simulink model "center_tapped_RL_high"  (R2022b)
settings: Solver=VariableStepAuto  StartTime=0.0  StopTime=00.1  RelTol=1e-3
libraries: spsCurrentMeasurementLib x3, spsVoltageMeasurementLib x3, spsDiodeLib x2, spsACVoltageSourceLib x1, spsLinearTransformerLib x1, spsSeriesRLCBranchLib x1, sps_lib x1
settings Model: Creator=mroun  LastModifiedBy=mroun

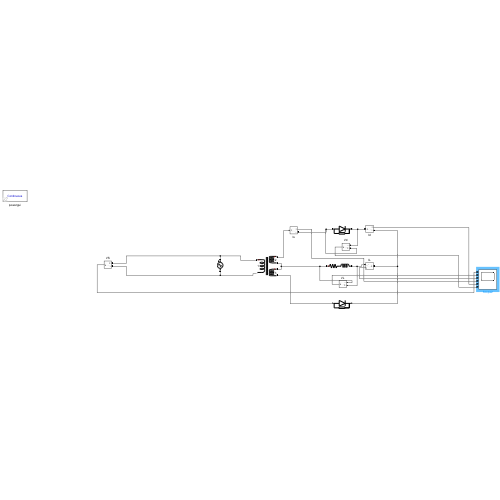
[thumbnail: Simulink's stored preview of the top-level diagram]
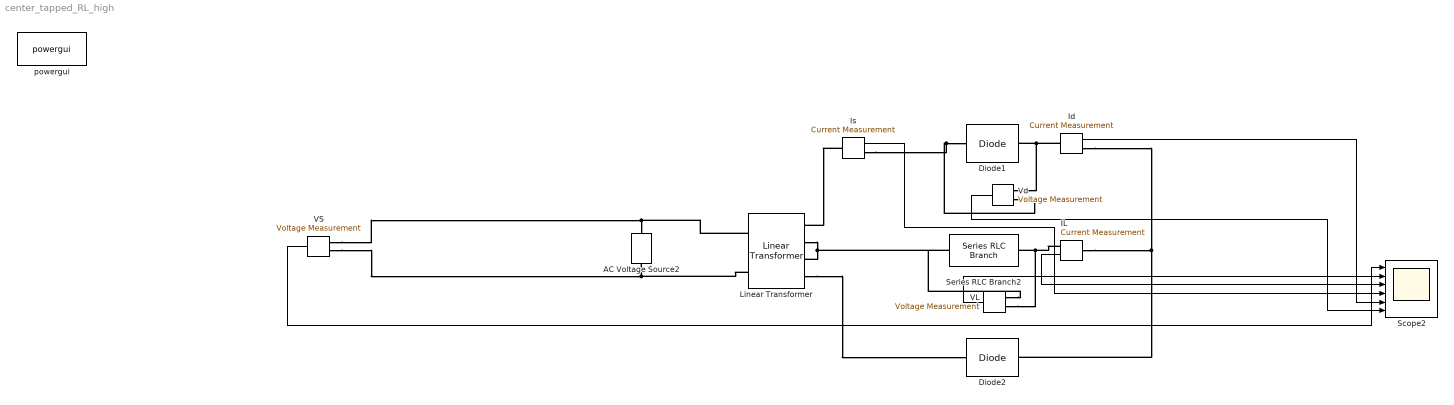
== system center_tapped_RL_high ==
  AC Voltage Source2 : spsACVoltageSourceLib/AC Voltage Source  Amplitude=200  Phase=0  Frequency=50  SampleTime=0  Measurements=None  BusType=swing  Pref=10e3  Qref=0  Qmin=-inf  Qmax=+inf
  Diode1 : spsDiodeLib/Diode  Ron=0.001  Lon=0  Vf=0.8  IC=0  UseSnubber=0  Rs=500  Cs=250e-9  Measurements=off
  Diode2 : spsDiodeLib/Diode  Ron=0.001  Lon=0  Vf=0.8  IC=0  UseSnubber=0  Rs=500  Cs=250e-9  Measurements=off
  IL : spsCurrentMeasurementLib/Current Measurement  PhasorSimulation=off  OutputType=Complex  PSBequivalent=0
  Id : spsCurrentMeasurementLib/Current Measurement  PhasorSimulation=off  OutputType=Complex  PSBequivalent=0
  Is : spsCurrentMeasurementLib/Current Measurement  PhasorSimulation=off  OutputType=Complex  PSBequivalent=0
  Linear Transformer : spsLinearTransformerLib/Linear Transformer  UNITS=pu  NominalPower=[ 1e3 50 ]  winding1="[ 200  0.002  0.08 ]"  winding2="[ 100  0.002  0.08 ]"  ThreeWindings=on  winding3=[ 100 0.002 0.08 ]  RmLm=[ 2 1 ]  Measurements=None  DataType=off
  Scope2 : Scope  NumInputPorts=6
  Series RLC Branch2 : spsSeriesRLCBranchLib/Series RLC Branch  LConnTagsString=__new0  RConnTagsString=__new0  BranchType=RL  Resistance=10  Inductance=1  SetiL0=off  InitialCurrent=2  Capacitance=1e-6  Setx0=off  InitialVoltage=0  Measurements=None
  VL : spsVoltageMeasurementLib/Voltage Measurement  PhasorSimulation=off  OutputType=Complex  PSBequivalent=0
  VS : spsVoltageMeasurementLib/Voltage Measurement  PhasorSimulation=off  OutputType=Complex  PSBequivalent=0
  Vd : spsVoltageMeasurementLib/Voltage Measurement  PhasorSimulation=off  OutputType=Complex  PSBequivalent=0
  powergui : sps_lib/powergui  Priority=1  SimulationMode=Continuous  SampleTime=50e-6  frequency=60  Iterations=50  frequencyindice=50  Pbase=100e6  ErrMax=1e-4  UnitsV=kV  UnitsW=MW  buscounter=0  FunctionMessages=off  echomessages=off  EnableUseOfTLC=off  CurrentSourceSwitches=off  DisableSnubberDevices=off  DisableRonSwitches=off  DisableVfSwitches=off  DisplayEquations=off  AutomaticDiscreteSolvers=off  SolverType=Tustin/Backward Euler (TBE)  Interpol=off  ExternalGateDelay=off  methode=off  Ts=100  x0status=blocks  SPID=on  SwTol=0  HookPort=off  NonlinearTolerance=1e-4  nMaxIteration=100  ContinueOnMaxIteration=off  RestoreLinks=warning  ResistiveCurrentMeasurement=off  Frange=[0:2:500]  Ylog=off  Xlog=on  ShowGrid=off  save=off  variable=ZData  structure=0  ZoomFFT=off  StartTime=0.0  cycles=1  DisplayStyle=1  fundamental=60  FreqAxis=off  MaxFrequency=1000  frequencyindicesteady=1  RmsSteady=1  display=off
  wires:
  VL/1 -> Scope2/2
  IL/1 -> Scope2/3
  Vd/1 -> Scope2/6
  Id/1 -> Scope2/5
  VS/1 -> Scope2/1
  Is/1 -> Scope2/4
  connections:
  VS/LConn1 -- Linear Transformer/LConn1 -- AC Voltage Source2/RConn1
  VS/LConn2 -- Linear Transformer/LConn2 -- AC Voltage Source2/LConn1
  Vd/LConn1 -- Is/RConn1 -- Diode1/LConn1
  Linear Transformer/RConn4 -- Diode2/LConn1
  Id/RConn1 -- Diode2/RConn1 -- IL/LConn1
  IL/RConn1 -- VL/LConn1 -- Series RLC Branch2/RConn1
  Id/LConn1 -- Vd/LConn2 -- Diode1/RConn1
  Linear Transformer/RConn2 -- VL/LConn2 -- Series RLC Branch2/LConn1 -- Linear Transformer/RConn3
  Is/LConn1 -- Linear Transformer/RConn1
